simulink subsystem "BatteryForTest2_refsub"  (R2022a)
settings: Solver=VariableStepAuto  StartTime=0.0  StopTime=10.0  RelTol=1e-3
undefined symbols (not defined in the file): Minus, Plus, testharness
libraries: fl_lib x8, nesl_utility x5
settings Model: Creator=isaacito  LastModifiedBy=isaacito
settings SolverCC: AlgebraicLoopSolver=TrustRegion
settings DebuggingCC: UnconnectedInputMsg=warning  UnconnectedOutputMsg=warning  UnconnectedLineMsg=warning  SFMachineParentedDataDiag=warning
settings RTWCC: DLArmComputeVersion=19.05

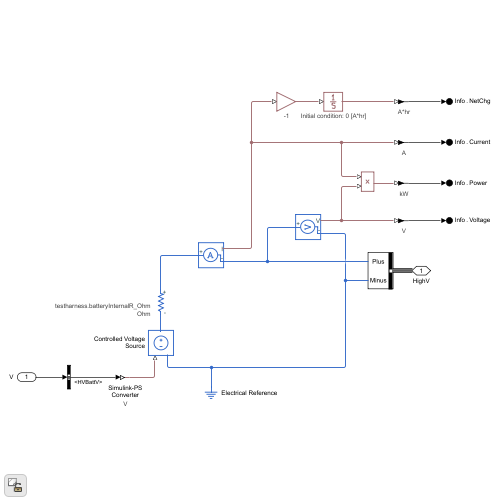
[thumbnail: Simulink's stored preview of the top-level diagram]
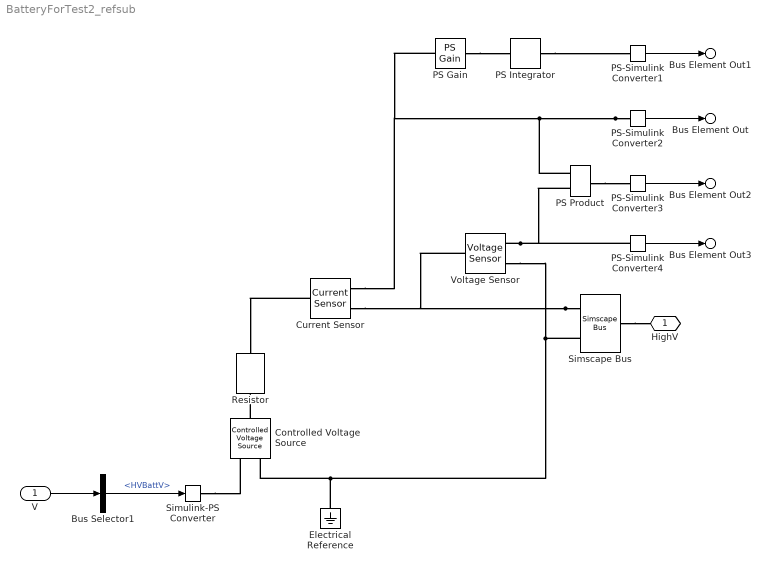
== system BatteryForTest2_refsub ==
  V : Inport
  Bus Selector1 : BusSelector  OutputSignals=HVBattV
  Controlled Voltage Source : fl_lib/Electrical/Electrical Sources/Controlled Voltage Source
      settings: SourceProductBaseCode=PW,SS,VE
  Current Sensor : fl_lib/Electrical/Electrical Sensors/Current Sensor
      settings: SourceProductBaseCode=PW,SS,VE
  Electrical Reference : fl_lib/Electrical/Electrical Elements/Electrical Reference
      settings: SourceProductBaseCode=PW,SS,VE
  PS Gain : fl_lib/Physical Signals/Functions/PS Gain  gain=-1
      settings: AttributesFormatString=%<gain>  SourceProductBaseCode=PW,SS,VE
  PS Integrator : fl_lib/Physical Signals/Linear Operators/PS Integrator  reset_method=foundation.enum.IntegratorResetSpec.None  initial_condition_spec=foundation.enum.IntegratorICSpec.Internal  x0=0 A*hr
      settings: AttributesFormatString=Initial condition: %<x0> [%<x0_unit>]  SourceProductBaseCode=PW,SS,VE
  PS Product : fl_lib/Physical Signals/Functions/PS Product
      settings: SourceProductBaseCode=PW,SS,VE
  PS-Simulink Converter1 : nesl_utility/PS-Simulink Converter  PhysicalDomain=network_engine_domain  SubClassName=ps_output  LeftPortType=input  RightPortType=output  PseudoPeriodic=off  Frequencies=[]  VectorFormat=1-D array  Unit=A*hr  AffineConversion=off
      settings: SourceProductBaseCode=SS,PW,VE
  PS-Simulink Converter2 : nesl_utility/PS-Simulink Converter  PhysicalDomain=network_engine_domain  SubClassName=ps_output  LeftPortType=input  RightPortType=output  PseudoPeriodic=off  Frequencies=[]  VectorFormat=1-D array  Unit=A  AffineConversion=off
      settings: SourceProductBaseCode=SS,PW,VE
  PS-Simulink Converter3 : nesl_utility/PS-Simulink Converter  PhysicalDomain=network_engine_domain  SubClassName=ps_output  LeftPortType=input  RightPortType=output  PseudoPeriodic=off  Frequencies=[]  VectorFormat=1-D array  Unit=kW  AffineConversion=off
      settings: SourceProductBaseCode=SS,PW,VE
  PS-Simulink Converter4 : nesl_utility/PS-Simulink Converter  PhysicalDomain=network_engine_domain  SubClassName=ps_output  LeftPortType=input  RightPortType=output  PseudoPeriodic=off  Frequencies=[]  VectorFormat=1-D array  Unit=V  AffineConversion=off
      settings: SourceProductBaseCode=SS,PW,VE
  Resistor : fl_lib/Electrical/Electrical Elements/Resistor  R=testharness.batteryInternalR_Ohm Ohm  i_specify=off  i_priority=None  i=0 A  i_nominal_specify=off  i_nominal_unit=A  i_nominal_value=1  v_specify=off  v_priority=None  v=0 V  v_nominal_specify=off  v_nominal_unit=V  v_nominal_value=1
      settings: SourceProductBaseCode=PW,SS,VE
      settings: AttributesFormatString=|
      | %<R>
      | %<R_unit>
  Simscape Bus : SimscapeBus  HierarchyStrings=Plus;Minus
  Simulink-PS Converter : nesl_utility/Simulink-PS Converter  PhysicalDomain=network_engine_domain  SubClassName=ps_input  LeftPortType=input  RightPortType=output  PseudoPeriodic=off  Frequencies=[]  NoiseDistribution=none  NoiseParameters=[]  Unit=V  AffineConversion=off  FilteringAndDerivatives=provide  SimscapeFilterOrder=1  InputFilterTimeConstant=0.001  UdotUserProvided=0
      settings: SourceProductBaseCode=SS,PW,VE
  Voltage Sensor : fl_lib/Electrical/Electrical Sensors/Voltage Sensor
      settings: SourceProductBaseCode=PW,SS,VE
  HighV : PMIOPort  Side=Right
  Bus Element Out : Outport  PortName=Info  Element=Current
  Bus Element Out1 : Outport  PortName=Info  Element=NetChg
  Bus Element Out2 : Outport  PortName=Info  Element=Power
  Bus Element Out3 : Outport  PortName=Info  Element=Voltage
  wires:
  PS-Simulink Converter1/1 -> Bus Element Out1/1
  PS-Simulink Converter4/1 -> Bus Element Out3/1
  PS-Simulink Converter3/1 -> Bus Element Out2/1
  PS-Simulink Converter2/1 -> Bus Element Out/1
  Bus Selector1/1 -> Simulink-PS Converter/1  "<HVBattV>"
  V/1 -> Bus Selector1/1
  connections:
  Voltage Sensor/RConn2 -- Controlled Voltage Source/RConn2 -- Electrical Reference/LConn1 -- Simscape Bus/LConn2
  Controlled Voltage Source/LConn1 -- Resistor/RConn1
  Simulink-PS Converter/RConn1 -- Controlled Voltage Source/RConn1
  Voltage Sensor/RConn1 -- PS-Simulink Converter4/LConn1 -- PS Product/LConn2
  Simscape Bus/LConn1 -- Current Sensor/RConn2 -- Voltage Sensor/LConn1
  PS-Simulink Converter2/LConn1 -- Current Sensor/RConn1 -- PS Gain/LConn1 -- PS Product/LConn1
  Simscape Bus/RConn1 -- HighV/RConn1
  Current Sensor/LConn1 -- Resistor/LConn1
  PS Integrator/RConn1 -- PS-Simulink Converter1/LConn1
  PS Product/RConn1 -- PS-Simulink Converter3/LConn1
  PS Gain/RConn1 -- PS Integrator/LConn1
